simulink model "Generador_2023"  (R2023b)
settings: Solver=VariableStepAuto  StartTime=0.0  StopTime=2  RelTol=1e-3
InitFcn:
  | clear; clc;
  | 
  | % Constantes del modelo
  | R=10; L=0.1; K=1500; Km=110; B=4500; J=1900; rm=1;
  | 
  | %Punto de equilibrio
  | vqo = 1;
  | wo = ((800*(vqo^2) + 1500*vqo)*rm)/(Km*K/R + B + rm*(800*vqo*rm - 1500));
  | io = K*wo/R;
  | Vo = K*wo;
StopFcn:
  | %Plotea datos
  | figure(1);
  | subplot(2,2,1), plot(t, vq);
  | grid on; xlabel('t'); ylabel('vq');
  | title('Velocidad caudal (m/s)');
  | 
  | subplot(2,2,2), plot(t, V);
  | grid on; xlabel('t'); ylabel('V');
  | title ('Tensión (V)');
  | 
  | subplot(2,2,3), plot(t, w);
  | grid on; xlabel('t'); ylabel('w');
  | title('Velocidad generador (rad/s)');
  | 
  | subplot(2,2,4), plot(t, in);
  | grid on; xlabel('t'); ylabel('i');
  | title('Intensidad (A)');
settings Model: Creator=rpiza  LastModifiedBy=rpiza
settings DataIOCC: SaveTime=off  ReturnWorkspaceOutputs=off

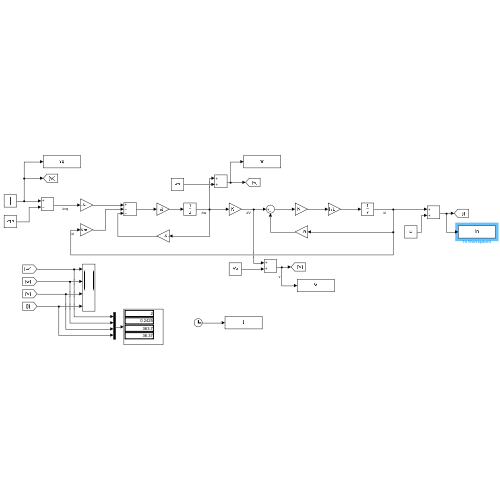
[thumbnail: Simulink's stored preview of the top-level diagram]
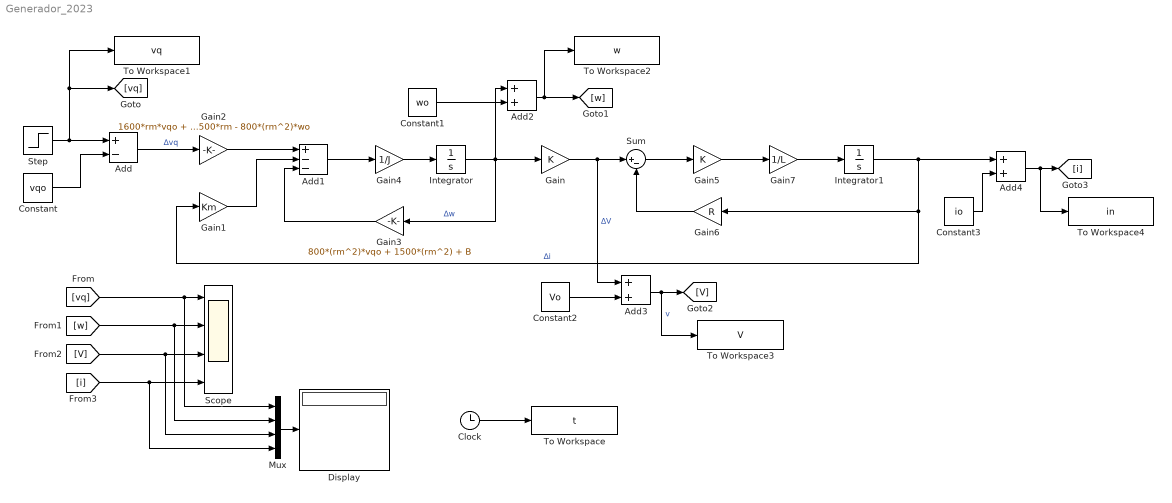
== system Generador_2023 ==
  Add : Sum  Inputs=+-
  Add1 : Sum  Inputs=+--
  Add2 : Sum
  Add3 : Sum
  Add4 : Sum
  Clock : Clock
  Constant : Constant  Value=vqo
  Constant1 : Constant  Value=wo
  Constant2 : Constant  Value=Vo
  Constant3 : Constant  Value=io
  Display : Display
  Gain : Gain  Gain=K
  Gain1 : Gain  Gain=Km
  Gain2 : Gain  Gain=1600*rm*vqo + 1500*rm - 800*(rm^2)*wo
  Gain3 : Gain  Gain=800*(rm^2)*vqo + 1500*(rm^2) + B
  Gain4 : Gain  Gain=1/J
  Gain5 : Gain  Gain=K
  Gain6 : Gain  Gain=R
  Gain7 : Gain  Gain=1/L
  Integrator : Integrator
  Integrator1 : Integrator
  Mux : Mux
  Scope : Scope  NumInputPorts=4
  Step : Step  Before=vqo  After=2  SampleTime=0
  Sum : Sum  Inputs=|+-
  To Workspace : ToWorkspace  VariableName=t  SampleTime=-1
  To Workspace1 : ToWorkspace  VariableName=vq  SampleTime=-1
  To Workspace2 : ToWorkspace  VariableName=w  SampleTime=-1
  To Workspace3 : ToWorkspace  VariableName=V  SampleTime=-1
  To Workspace4 : ToWorkspace  VariableName=in  SampleTime=-1
  wires:
  Clock/1 -> To Workspace/1
  Step/1 -> [vq], To Workspace1/1, Add/1
  Add/1 -> Gain2/1  "∆vq"
  Constant/1 -> Add/2
  Gain4/1 -> Integrator/1
  Gain2/1 -> Add1/1
  Integrator/1 -> Gain3/1, Add2/1, Gain/1  "∆w"
  Gain1/1 -> Add1/2
  Add1/1 -> Gain4/1
  Gain3/1 -> Add1/3
  Gain7/1 -> Integrator1/1
  Gain6/1 -> Sum/2
  Integrator1/1 -> Add4/1, Gain6/1, Gain1/1  "∆i"
  Gain5/1 -> Gain7/1
  Gain/1 -> Add3/1, Sum/1  "∆V"
  Sum/1 -> Gain5/1
  Constant1/1 -> Add2/2
  Add2/1 -> To Workspace2/1, [w]
  Constant2/1 -> Add3/2
  Add3/1 -> To Workspace3/1, [V]  "v"
  Constant3/1 -> Add4/2
  Add4/1 -> To Workspace4/1, [i]
  [vq] -> Mux/1, Scope/1
  [w] -> Mux/2, Scope/2
  [V] -> Mux/3, Scope/3
  [i] -> Mux/4, Scope/4
  Mux/1 -> Display/1
